simulink model "sampleModel1576"  (R2023a)
settings: Solver=VariableStepAuto  StartTime=0.0  StopTime=10.0  RelTol=1e-3
libraries: hdlsllib x6, simulink x4
settings Model: Creator=user1  LastModifiedBy=user1

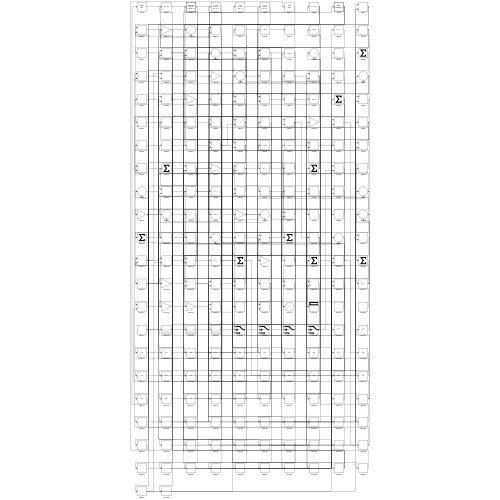
[thumbnail: Simulink's stored preview of the top-level diagram]
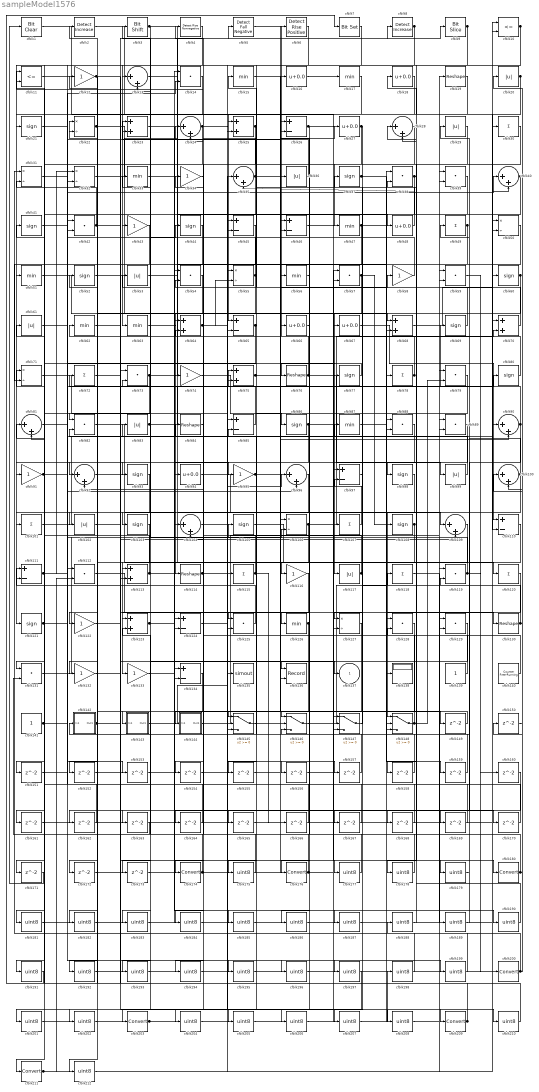
== system sampleModel1576 ==
  cfblk1 : simulink/Logic and Bit Operations/Bit Clear  iBit=0
      settings: LibrarySourceBlock=|
      | hdlsllib/Logic and Bit
      | Operations/Bit Clear
  cfblk10 : RelationalOperator  Operator=<=  OutDataTypeStr=boolean  InputSameDT=off
  cfblk{13,24,28,35,40,81,90,92,96,100,104,109} (12 alike) : Sum  Inputs=|++
  cfblk{30,49,72,78,101,107,115,118,120} (9 alike) : Sum  Inputs=+
  cfblk{20,29,36,53,61,83,99,102,117} (9 alike) : Abs  SaturateOnIntegerOverflow=off
  cfblk{21,37,41,44,52,60,69,77,80,86,93,98,103,105,108,121} (16 alike) : Signum
  cfblk{22,31..32,50,55,71,106,127} (8 alike) : Product  Inputs=*/  RndMeth=Zero  SaturateOnIntegerOverflow=on
  cfblk11 : RelationalOperator  Operator=<=  OutDataTypeStr=boolean  InputSameDT=off
  cfblk{26,45..46,65,85,97,110..111,124,134} (10 alike) : Sum  Inputs=+-
  cfblk{14,38..39,42,54,57,59,73,79,82,88..89,112,119,125,128..129,131} (18 alike) : DotProduct  OutDataTypeStr=Inherit: Inherit via internal rule
  cfblk{23,25,64,68,70,75,113,123} (8 alike) : Sum
  cfblk{19,76,84,114,130} (5 alike) : Reshape
  cfblk{12,34,43,58,74,91,95,116,122,132..133} (11 alike) : Gain
  cfblk{15,17,33,47,51,56,62..63,87,126} (10 alike) : MinMax
  cfblk135 : ToWorkspace  VariableName=simout  SaveFormat=Timeseries  SampleTime=-1
  cfblk136 : Record  FileSettingsInternal="{\"entries\":[{\"content\":{\"excelSettings\":{\"content\":{},\"type\":\"Streamout.ExcelSettings\"}},\"type\":\"Streamout.FileSettingStorage\",\"uuid\":\"\"}],\"packageUris\":[\"http:\\/\\/schema.mathworks.com\\/mf0\\/streamout_blocks\\/R2020a\"],\"version\":\"1.0\"}"  Layout=[1 1]  SignalsInternal="{\"entries\":[{\"content\":{\"signals\":[{\"content\":{\"blockPath\":[],\"dimensions\":[1],\"domain\":\"\",\"lineColor\":\"#a2142f\",\"plots\":[1],\"port\":1,\"signalID\":1913,\"signalName\":\"XY Graph:1\"},\"type\":\"RecordBlkView.Signal\",\"uuid\":\"\"},{\"content\":{\"blockPath\":[],\"dimensions\":[1],\"domain\":\"\",\"lineColor\":\"#139fff\",\"plots\":[1],\"port\":2,\"signalID\":1916,\"signalName\":\"XY Graph:2\"},\"type\":\"RecordBlkView.Signal\",\"uuid\":\"\"}]},\"type\":\"RecordBlkView.InputSignals\",\"uuid\":\"\"}],\"packageUris\":[\"http:\\/\\/schema.mathworks.com\\/mf0\\/streamout_blocks\\/R2020a\"],\"version\":\"1.0\"}"  VisualizationBindings="{\"xyplotplugin\":{\"info\":[{\"series\":[{\"bindingParametersList\":[{\"parameter\":\"X-Axis\",\"signalID\":1913,\"signalName\":\"XY Graph:1\"},{\"parameter\":\"Y-Axis\",\"signalID\":1916,\"signalName\":\"XY Graph:2\"}],\"seriesID\":59425}],\"subplotID\":1}]}}"  CompatibilityTag=XY  st=-1
  cfblk138 : Display
  cfblk139 : Constant  SampleTime=-1
  cfblk140 : hdlsllib/Sources/Counter Free-Running  NumBits=16  tsamp=-1
  cfblk141 : Constant  SampleTime=-1
  cfblk142 : Subsystem
      settings: LibrarySourceBlock=|
      | hdlsllib/Ports &
      | Subsystems/Subsystem
  cfblk143 : Subsystem
      settings: LibrarySourceBlock=|
      | hdlsllib/Ports &
      | Subsystems/Subsystem
  cfblk144 : Subsystem
      settings: LibrarySourceBlock=|
      | hdlsllib/Ports &
      | Subsystems/Subsystem
  cfblk{145..148} (4 alike) : Switch  SaturateOnIntegerOverflow=off  InputSameDT=off
  cfblk{149..173} (25 alike) : Delay  SampleTime=1
  cfblk{16,18,27,48,66..67,94} (7 alike) : Bias  Bias=0.0  SaturateOnIntegerOverflow=off
  cfblk{174,176,180,200,203,209,211} (7 alike) : DataTypeConversion  SaturateOnIntegerOverflow=off  RndMeth=Floor
  cfblk{175,177..179,181..199,201..202,204..208,210,212} (32 alike) : DataTypeConversion  OutDataTypeStr=uint8  SaturateOnIntegerOverflow=off  RndMeth=Floor
  cfblk2 : simulink/Logic and Bit Operations/Detect Increase  vinit=0.0  OutDataTypeStr=boolean
      settings: LibrarySourceBlock=|
      | hdlsllib/Logic and Bit
      | Operations/Detect
      | Increase
  cfblk3 : hdlsllib/Logic and Bit Operations/Bit Shift  mode=Shift Left Logical  N=0
  cfblk4 : hdlsllib/Logic and Bit Operations/Detect Rise Nonnegative  vinit=0  OutDataTypeStr=boolean
  cfblk5 : hdlsllib/Logic and Bit Operations/Detect Fall Negative  vinit=0  OutDataTypeStr=boolean
  cfblk6 : hdlsllib/Logic and Bit Operations/Detect Rise Positive  vinit=0  OutDataTypeStr=boolean
  cfblk7 : simulink/Logic and Bit Operations/Bit Set  iBit=0
      settings: LibrarySourceBlock=|
      | hdlsllib/Logic and Bit
      | Operations/Bit Set
  cfblk8 : simulink/Logic and Bit Operations/Detect Increase  vinit=0.0  OutDataTypeStr=boolean
      settings: LibrarySourceBlock=|
      | hdlsllib/Logic and Bit
      | Operations/Detect
      | Increase
  cfblk9 : hdlsllib/Logic and Bit Operations/Bit Slice  lidx=7  ridx=0
  cfblk137 : Outport  VectorParamsAs1DForOutWhenUnconnected=off
  wires:
  cfblk28/1 -> cfblk47/1
  cfblk86/1 -> cfblk161/1, cfblk179/1
  cfblk55/1 -> cfblk104/2, cfblk3/1, cfblk204/1
  cfblk8/1 -> cfblk121/1, cfblk65/2, cfblk113/1
  cfblk130/1 -> cfblk20/1, cfblk87/1
  cfblk39/1 -> cfblk203/1
  cfblk67/1 -> cfblk110/1
  cfblk10/1 -> cfblk65/1, cfblk175/1
  cfblk33/1 -> cfblk48/1
  cfblk14/1 -> cfblk21/1
  cfblk84/1 -> cfblk174/1
  cfblk20/1 -> cfblk110/2, cfblk25/2
  cfblk131/1 -> cfblk105/1
  cfblk9/1 -> cfblk63/1, cfblk13/1, cfblk32/2
  cfblk3/1 -> cfblk116/1, cfblk103/1
  cfblk78/1 -> cfblk6/1, cfblk13/2
  cfblk22/1 -> cfblk117/1, cfblk127/2
  cfblk56/1 -> cfblk176/1
  cfblk36/1 -> cfblk23/1
  cfblk73/1 -> cfblk5/1, cfblk136/2, cfblk171/1, cfblk182/1
  cfblk26/1 -> cfblk146/1, cfblk68/2
  cfblk115/1 -> cfblk82/2, cfblk166/1
  cfblk60/1 -> cfblk114/1, cfblk158/1
  cfblk40/1 -> cfblk125/1, cfblk152/1
  cfblk32/1 -> cfblk8/1
  cfblk53/1 -> cfblk109/1
  cfblk66/1 -> cfblk26/1
  cfblk47/1 -> cfblk159/1, cfblk193/1
  cfblk5/1 -> cfblk46/1
  cfblk90/1 -> cfblk12/1, cfblk169/1
  cfblk44/1 -> cfblk82/1
  cfblk110/1 -> cfblk142/1(In1)
  cfblk139/1 -> cfblk18/1
  cfblk92/1 -> cfblk104/1
  cfblk106/1 -> cfblk70/2, cfblk184/1
  cfblk76/1 -> cfblk98/1, cfblk64/2
  cfblk141/1 -> cfblk26/2, cfblk96/2
  cfblk101/1 -> cfblk10/1
  cfblk103/1 -> cfblk122/1
  cfblk121/1 -> cfblk75/1, cfblk44/1, cfblk14/2
  cfblk82/1 -> cfblk120/1
  cfblk74/1 -> cfblk86/1
  cfblk49/1 -> cfblk101/1, cfblk71/2
  cfblk77/1 -> cfblk76/1
  cfblk35/1 -> cfblk131/1, cfblk147/2, cfblk11/2
  cfblk126/1 -> cfblk136/1, cfblk164/1
  cfblk63/1 -> cfblk94/1
  cfblk30/1 -> cfblk211/1
  cfblk4/1 -> cfblk91/1
  cfblk2/1 -> cfblk107/1
  cfblk37/1 -> cfblk99/1, cfblk207/1
  cfblk87/1 -> cfblk80/1
  cfblk108/1 -> cfblk133/1, cfblk205/1
  cfblk120/1 -> cfblk148/1
  cfblk38/1 -> cfblk35/2, cfblk68/1, cfblk125/2
  cfblk18/1 -> cfblk46/2
  cfblk68/1 -> cfblk10/2
  cfblk24/1 -> cfblk51/1, cfblk210/1
  cfblk75/1 -> cfblk27/1, cfblk165/1
  cfblk123/1 -> cfblk168/1, cfblk185/1
  cfblk114/1 -> cfblk156/1, cfblk157/1
  cfblk61/1 -> cfblk40/1
  cfblk54/1 -> cfblk92/1
  cfblk146/1 -> cfblk38/1
  cfblk97/1 -> cfblk37/1
  cfblk117/1 -> cfblk92/2, cfblk167/1
  cfblk105/1 -> cfblk147/1
  cfblk94/1 -> cfblk138/1
  cfblk69/1 -> cfblk15/1
  cfblk19/1 -> cfblk143/1(In1)
  cfblk15/1 -> cfblk36/1
  cfblk147/1 -> cfblk97/2
  cfblk64/1 -> cfblk55/2, cfblk187/1
  cfblk27/1 -> cfblk127/1, cfblk113/2
  cfblk111/1 -> cfblk81/1, cfblk106/2, cfblk32/1
  cfblk144/1(Out1) -> cfblk19/1
  cfblk100/1 -> cfblk49/1, cfblk172/1
  cfblk143/1(Out1) -> cfblk85/1
  cfblk25/1 -> cfblk74/1, cfblk45/1
  cfblk6/1 -> cfblk43/1
  cfblk58/1 -> cfblk33/1
  cfblk80/1 -> cfblk22/1
  cfblk119/1 -> cfblk28/1, cfblk53/1, cfblk160/1
  cfblk112/1 -> cfblk130/1
  cfblk116/1 -> cfblk123/1
  cfblk142/1(Out1) -> cfblk75/2, cfblk52/1
  cfblk72/1 -> cfblk209/1
  cfblk43/1 -> cfblk132/1
  cfblk113/1 -> cfblk71/1, cfblk126/1
  cfblk12/1 -> cfblk102/1, cfblk109/2
  cfblk57/1 -> cfblk144/1(In1), cfblk64/1, cfblk108/1
  cfblk99/1 -> cfblk4/1
  cfblk98/1 -> cfblk148/2
  cfblk145/1 -> cfblk58/1
  cfblk16/1 -> cfblk17/1
  cfblk52/1 -> cfblk115/1
  cfblk21/1 -> cfblk42/2
  cfblk59/1 -> cfblk200/1
  cfblk11/1 -> cfblk25/1
  cfblk13/1 -> cfblk148/3
  cfblk104/1 -> cfblk96/1
  cfblk1/1 -> cfblk57/2
  cfblk83/1 -> cfblk69/1, cfblk95/1
  cfblk65/1 -> cfblk145/2, cfblk181/1
  cfblk122/1 -> cfblk9/1
  cfblk41/1 -> cfblk77/1
  cfblk42/1 -> cfblk11/1, cfblk134/2
  cfblk124/1 -> cfblk180/1
  cfblk70/1 -> cfblk24/1
  cfblk125/1 -> cfblk111/1
  cfblk107/1 -> cfblk66/1
  cfblk85/1 -> cfblk2/1
  cfblk51/1 -> cfblk135/1
  cfblk45/1 -> cfblk93/1
  cfblk71/1 -> cfblk145/3
  cfblk148/1 -> cfblk34/1, cfblk79/2
  cfblk91/1 -> cfblk83/1, cfblk73/2
  cfblk95/1 -> cfblk90/2, cfblk137/1
  cfblk140/1 -> cfblk28/2
  cfblk7/1 -> cfblk81/2
  cfblk48/1 -> cfblk23/2
  cfblk23/1 -> cfblk149/1
  cfblk149/1 -> cfblk145/1
  cfblk150/1 -> cfblk100/2
  cfblk96/1 -> cfblk151/1
  cfblk152/1 -> cfblk35/1
  cfblk81/1 -> cfblk153/1
  cfblk153/1 -> cfblk146/2
  cfblk34/1 -> cfblk154/1
  cfblk79/1 -> cfblk155/1
  cfblk155/1 -> cfblk106/1
  cfblk156/1 -> cfblk97/1
  cfblk157/1 -> cfblk24/2
  cfblk158/1 -> cfblk146/3
  cfblk159/1 -> cfblk85/2
  cfblk161/1 -> cfblk70/1
  cfblk93/1 -> cfblk162/1
  cfblk162/1 -> cfblk42/1
  cfblk127/1 -> cfblk163/1
  cfblk163/1 -> cfblk131/2
  cfblk164/1 -> cfblk111/2
  cfblk165/1 -> cfblk40/2
  cfblk166/1 -> cfblk112/1
  cfblk167/1 -> cfblk134/1
  cfblk168/1 -> cfblk57/1
  cfblk169/1 -> cfblk55/1
  cfblk46/1 -> cfblk170/1
  cfblk170/1 -> cfblk38/2
  cfblk171/1 -> cfblk1/1
  cfblk172/1 -> cfblk147/3
  cfblk17/1 -> cfblk173/1
  cfblk173/1 -> cfblk16/1
  cfblk174/1 -> cfblk123/2, cfblk61/1
  cfblk175/1 -> cfblk84/1
  cfblk176/1 -> cfblk14/1, cfblk62/1
  cfblk132/1 -> cfblk177/1
  cfblk177/1 -> cfblk56/1
  cfblk29/1 -> cfblk178/1
  cfblk178/1 -> cfblk54/1
  cfblk179/1 -> cfblk29/1
  cfblk180/1 -> cfblk150/1, cfblk54/2
  cfblk181/1 -> cfblk124/1
  cfblk182/1 -> cfblk124/2
  cfblk129/1 -> cfblk183/1
  cfblk183/1 -> cfblk90/1
  cfblk184/1 -> cfblk129/1
  cfblk185/1 -> cfblk129/2
  cfblk128/1 -> cfblk186/1
  cfblk186/1 -> cfblk60/1
  cfblk187/1 -> cfblk128/1
  cfblk188/1 -> cfblk128/2
  cfblk118/1 -> cfblk189/1
  cfblk189/1 -> cfblk119/2
  cfblk133/1 -> cfblk190/1
  cfblk190/1 -> cfblk118/1
  cfblk88/1 -> cfblk191/1
  cfblk191/1 -> cfblk7/1
  cfblk109/1 -> cfblk192/1
  cfblk192/1 -> cfblk88/1
  cfblk193/1 -> cfblk88/2
  cfblk50/1 -> cfblk194/1
  cfblk194/1 -> cfblk119/1
  cfblk102/1 -> cfblk195/1
  cfblk195/1 -> cfblk50/1
  cfblk62/1 -> cfblk196/1
  cfblk196/1 -> cfblk50/2
  cfblk31/1 -> cfblk197/1
  cfblk198/1 -> cfblk31/1
  cfblk151/1 -> cfblk199/1
  cfblk199/1 -> cfblk31/2
  cfblk200/1 -> cfblk188/1, cfblk100/1
  cfblk197/1 -> cfblk201/1
  cfblk201/1 -> cfblk59/1
  cfblk160/1 -> cfblk202/1
  cfblk202/1 -> cfblk59/2
  cfblk203/1 -> cfblk67/1, cfblk78/1
  cfblk204/1 -> cfblk39/1
  cfblk205/1 -> cfblk39/2
  cfblk89/1 -> cfblk206/1
  cfblk206/1 -> cfblk198/1
  cfblk207/1 -> cfblk89/1
  cfblk154/1 -> cfblk208/1
  cfblk208/1 -> cfblk89/2
  cfblk209/1 -> cfblk22/2, cfblk73/1, cfblk41/1
  cfblk210/1 -> cfblk72/1
  cfblk211/1 -> cfblk45/2, cfblk79/1, cfblk112/2
  cfblk134/1 -> cfblk212/1
  cfblk212/1 -> cfblk30/1

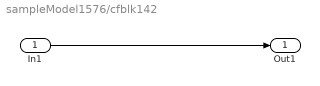
== system sampleModel1576/cfblk142 ==
  In1 : Inport
  Out1 : Outport
  wires:
  In1/1 -> Out1/1

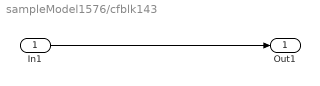
== system sampleModel1576/cfblk143 ==
  In1 : Inport
  Out1 : Outport
  wires:
  In1/1 -> Out1/1

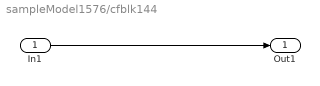
== system sampleModel1576/cfblk144 ==
  In1 : Inport
  Out1 : Outport
  wires:
  In1/1 -> Out1/1
